simulink subsystem "Lateral_Position_Control"  (R2021b)
settings: Solver=VariableStepAuto  StartTime=0.0  StopTime=10.0  RelTol=1e-3
undefined symbols (not defined in the file or in its folder): IC0, md, md0, PredictionHorizon, Ts, XRef, YawRef, YRef
libraries: simulink_extras x5, mpcadaslib x1, cstblocks x1
settings Model: Creator=gabep  LastModifiedBy=gabep

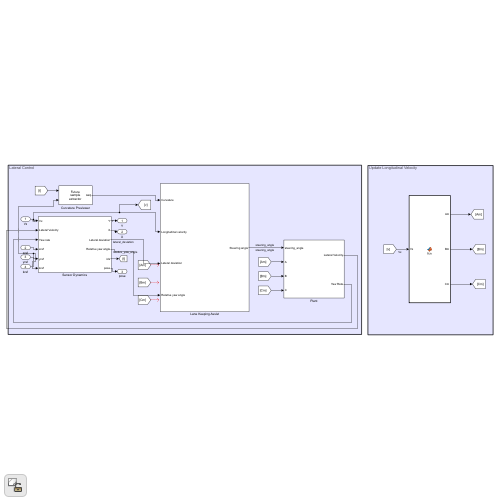
[thumbnail: Simulink's stored preview of the top-level diagram]
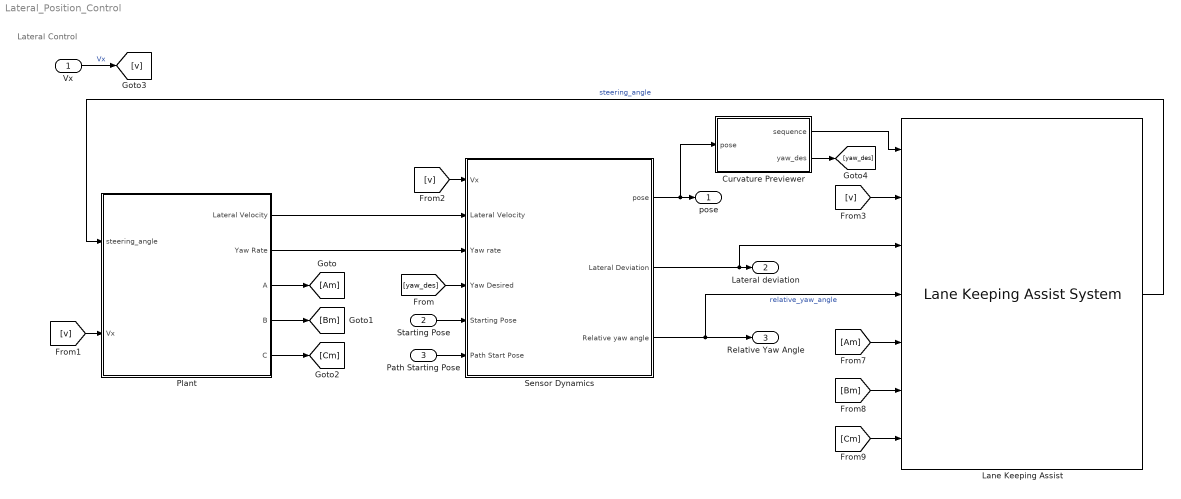
== system Lateral_Position_Control ==
  note: Lateral Control
  Vx : Inport
  Starting Pose : Inport  Port=2
  Path Starting Pose : Inport  Port=3
  Curvature Previewer : Subsystem  mask{signal=md, ts=Ts, steps=PredictionHorizon}
      mask prompts: signal "Signal name"; ts "Sampling time"; steps "Number of previewing steps"
      mask init:
      | ts = evalin('base',get_param(gcbh,'ts'));
      | signal = evalin('base',get_param(gcbh,'signal'));
      | steps = evalin('base',get_param(gcbh,'steps'));
      | data = mpc_previewer_maskinit(signal,ts);
      mask Display:
      | fprintf('Future\nsample\nextractor');
      | port_label('output', 1, 'seq')
      | %port_label('output', 2, '@t')
  Lane Keeping Assist : mpcadaslib/Lane Keeping Assist System  ModelType=Use vehicle model  VehicleMass=9053  VehicleYawInertia=52161  LengthToFront=2.7  LengthToRear=4.02  FrontTireStiffness=15000  RearTireStiffness=121000  EgoModelMatrixA=A  EgoModelMatrixB=B  EgoModelMatrixC=C  InitialLongVel=Vx0  TransportLag=0  MinSteering=u_min  umin_ext=off  MaxSteering=u_max  umax_ext=off  Ts=Ts  PredictionHorizon=PredictionHorizon  ControllerBehavior=0.500  suboptimal=off  maxiter=10  datatypeopt=double  optmode=off  trackmode=off
      settings: SourceProductBaseCode=MP
  Plant : Subsystem
  Sensor Dynamics : Subsystem
  pose : Outport
  Lateral deviation : Outport  Port=2
  Relative Yaw Angle : Outport  Port=3
  wires:
  Plant/2(Yaw Rate) -> Sensor Dynamics/3(Yaw rate)
  Plant/1(Lateral Velocity) -> Sensor Dynamics/2(Lateral Velocity)
  [Am] -> Lane Keeping Assist/5
  [Bm] -> Lane Keeping Assist/6
  [Cm] -> Lane Keeping Assist/7
  Sensor Dynamics/3(Relative yaw angle) -> Relative Yaw Angle/1, Lane Keeping Assist/4  "relative_yaw_angle"
  Lane Keeping Assist/1 -> Plant/1(steering_angle)  "steering_angle"
  Plant/3(A) -> [Am]
  Plant/5(C) -> [Cm]
  Plant/4(B) -> [Bm]
  Starting Pose/1 -> Sensor Dynamics/5(Starting Pose)
  Curvature Previewer/1(sequence) -> Lane Keeping Assist/1
  Path Starting Pose/1 -> Sensor Dynamics/6(Path Start Pose)
  Sensor Dynamics/1(pose) -> Curvature Previewer/1(pose), pose/1
  Vx/1 -> [v]  "Vx"
  [v] -> Sensor Dynamics/1(Vx)
  [v] -> Lane Keeping Assist/2
  [v] -> Plant/2(Vx)
  Curvature Previewer/2(yaw_des) -> [yaw_des]
  [yaw_des] -> Sensor Dynamics/4(Yaw Desired)
  Sensor Dynamics/2(Lateral Deviation) -> Lateral deviation/1, Lane Keeping Assist/3

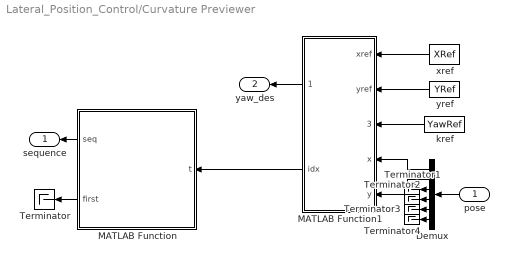
== system Lateral_Position_Control/Curvature Previewer ==
  pose : Inport
  Demux : Demux  Outputs=6
  MATLAB Function : MATLAB Function  TreatAsAtomicUnit=on
  MATLAB Function1 : MATLAB Function  TreatAsAtomicUnit=on
  Terminator{,1..4} (5 alike) : Terminator
  kref : Constant  Value=YawRef
  xref : Constant  Value=XRef
  yref : Constant  Value=YRef
  sequence : Outport  VectorParamsAs1DForOutWhenUnconnected=off
  yaw_des : Outport  Port=2
  wires:
  MATLAB Function1/1(yaw_des) -> yaw_des/1
  Demux/6 -> Terminator4/1
  Demux/5 -> Terminator3/1
  Demux/4 -> Terminator2/1
  Demux/3 -> Terminator1/1
  Demux/2 -> MATLAB Function1/5(y)
  Demux/1 -> MATLAB Function1/4(x)
  pose/1 -> Demux/1
  kref/1 -> MATLAB Function1/3(yawref)
  yref/1 -> MATLAB Function1/2(yref)
  xref/1 -> MATLAB Function1/1(xref)
  MATLAB Function1/2(idx) -> MATLAB Function/1(t)
  MATLAB Function/2(first) -> Terminator/1
  MATLAB Function/1(seq) -> sequence/1

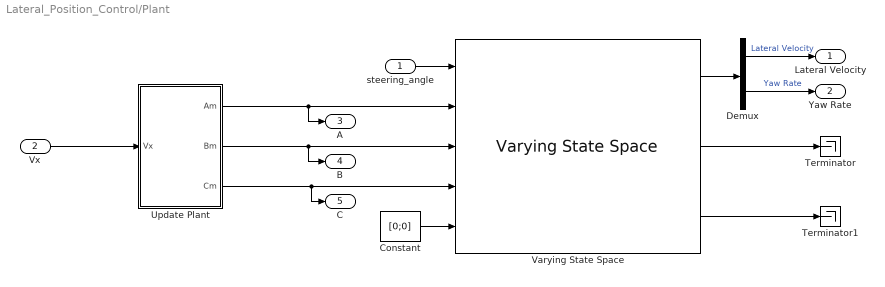
== system Lateral_Position_Control/Plant ==
  steering_angle : Inport
  Vx : Inport  Port=2
  Constant : Constant  Value=[0;0]
  Demux : Demux  Outputs=2
  Terminator : Terminator
  Terminator1 : Terminator
  Update Plant : MATLAB Function  TreatAsAtomicUnit=on
  Varying State Space : cstblocks/Linear Parameter Varying/Varying State Space  x0=0  xNames=''  OutputX=on  OutputDX=on
  Lateral Velocity : Outport
  Yaw Rate : Outport  Port=2
  A : Outport  Port=3
  B : Outport  Port=4
  C : Outport  Port=5
  wires:
  Vx/1 -> Update Plant/1(Vx)
  Update Plant/3(Cm) -> Varying State Space/4, C/1
  Update Plant/1(Am) -> Varying State Space/2, A/1
  Update Plant/2(Bm) -> Varying State Space/3, B/1
  Demux/2 -> Yaw Rate/1  "Yaw Rate"
  Varying State Space/1 -> Demux/1
  Varying State Space/2 -> Terminator/1
  Demux/1 -> Lateral Velocity/1  "Lateral Velocity"
  Varying State Space/3 -> Terminator1/1
  Constant/1 -> Varying State Space/5
  steering_angle/1 -> Varying State Space/1

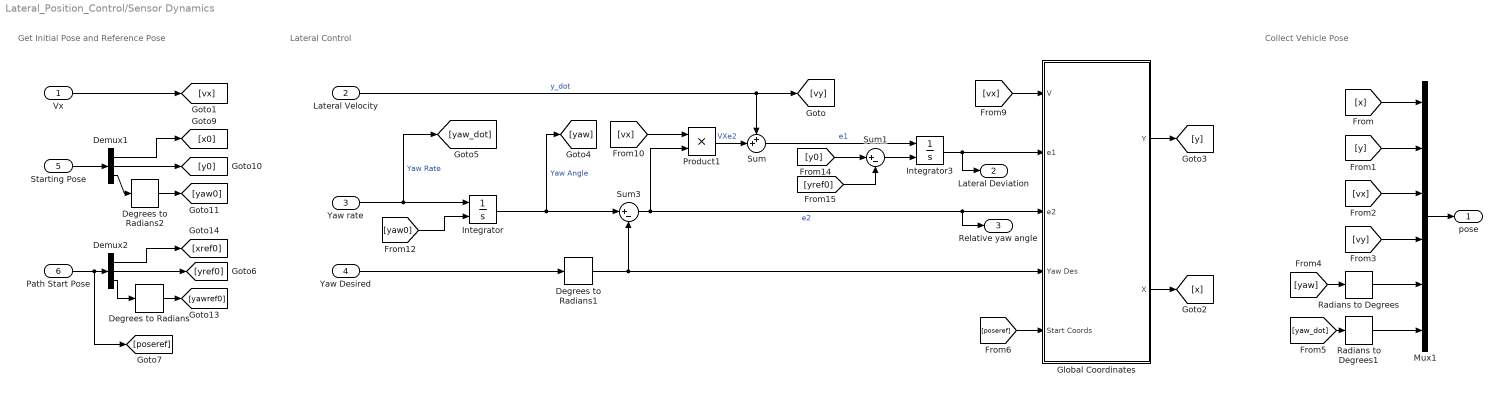
== system Lateral_Position_Control/Sensor Dynamics ==
  note: Get Initial Pose and Reference Pose
  note: Lateral Control
  note: Collect Vehicle Pose
  Vx : Inport
  Lateral Velocity : Inport  Port=2
  Yaw rate : Inport  Port=3
  Yaw Desired : Inport  Port=4
  Starting Pose : Inport  Port=5
  Path Start Pose : Inport  Port=6
  " Global Coordinates" : Subsystem
  Degrees to Radians : simulink_extras/Transformations/Degrees to Radians
  Degrees to Radians1 : simulink_extras/Transformations/Degrees to Radians
  Degrees to Radians2 : simulink_extras/Transformations/Degrees to Radians
  Demux1 : Demux  Outputs=3
  Demux2 : Demux  Outputs=3
  Integrator : Integrator  InitialConditionSource=external  InitialCondition=IC0.yaw_angle0
  Integrator3 : Integrator  InitialConditionSource=external  InitialCondition=IC0.y0 - md0.y(130)
  Mux1 : Mux  Inputs=6
  Product1 : Product
  Radians to Degrees : simulink_extras/Transformations/Radians to Degrees
  Radians to Degrees1 : simulink_extras/Transformations/Radians to Degrees
  Sum : Sum  Inputs=++|
  Sum1 : Sum  Inputs=|+-
  Sum3 : Sum  Inputs=|+-
  pose : Outport
  Lateral Deviation : Outport  Port=2
  Relative yaw angle : Outport  Port=3  VectorParamsAs1DForOutWhenUnconnected=off
  wires:
  Degrees to Radians1/1 -> " Global Coordinates"/4(Yaw Des), Sum3/2
  Yaw Desired/1 -> Degrees to Radians1/1
  Path Start Pose/1 -> Demux2/1, [poseref]
  Degrees to Radians2/1 -> [yaw0]
  Radians to Degrees/1 -> Mux1/5
  [vx] -> " Global Coordinates"/1(V)
  Degrees to Radians/1 -> [yawref0]
  [poseref] -> " Global Coordinates"/5(Start Coords)
  Demux2/2 -> [yref0]
  Demux2/1 -> [xref0]
  Sum1/1 -> Integrator3/2
  Sum/1 -> Integrator3/1  "e1"
  [yref0] -> Sum1/2
  [y0] -> Sum1/1
  [yaw0] -> Integrator/2
  [vx] -> Product1/1
  Vx/1 -> [vx]
  Demux2/3 -> Degrees to Radians/1
  Demux1/2 -> [y0]
  Demux1/3 -> Degrees to Radians2/1
  Demux1/1 -> [x0]
  Starting Pose/1 -> Demux1/1
  [yaw] -> Radians to Degrees/1
  [yaw_dot] -> Radians to Degrees1/1
  [vy] -> Mux1/4
  Mux1/1 -> pose/1
  [x] -> Mux1/1
  Radians to Degrees1/1 -> Mux1/6
  [vx] -> Mux1/3
  [y] -> Mux1/2
  Integrator3/1 -> " Global Coordinates"/2(e1), Lateral Deviation/1
  Sum3/1 -> " Global Coordinates"/3(e2), Relative yaw angle/1, Product1/2  "e2"
  " Global Coordinates"/2(X) -> [x]
  " Global Coordinates"/1(Y) -> [y]
  Product1/1 -> Sum/2  "VXe2"
  Lateral Velocity/1 -> [vy], Sum/1  "y_dot"
  Integrator/1 -> [yaw], Sum3/1  "Yaw Angle"
  Yaw rate/1 -> Integrator/1, [yaw_dot]  "Yaw Rate"

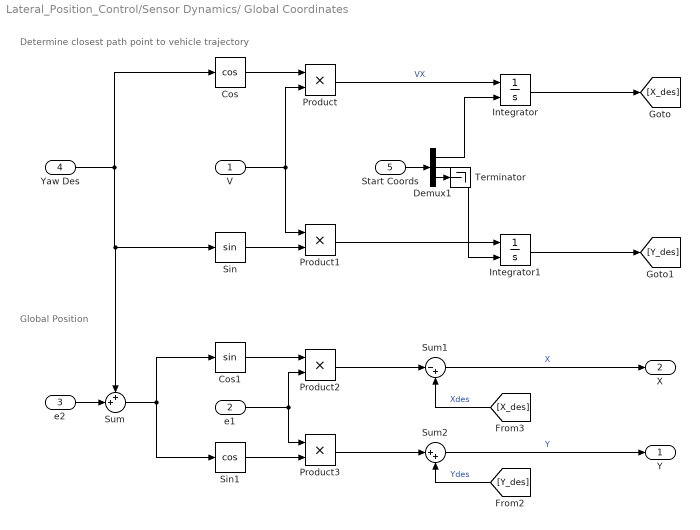
== system Lateral_Position_Control/Sensor Dynamics/ Global Coordinates ==
  note: Global Position
  note: Determine closest path point to vehicle trajectory
  V : Inport
  e1 : Inport  Port=2
  e2 : Inport  Port=3
  Yaw Des : Inport  Port=4
  Start Coords : Inport  Port=5
  Cos : Trigonometry  Operator=cos
  Cos1 : Trigonometry
  Demux1 : Demux  Outputs=3
  Integrator : Integrator  InitialConditionSource=external  InitialCondition=md0.x(130)
  Integrator1 : Integrator  InitialConditionSource=external  InitialCondition=md0.y(130)
  Product{,1..3} (4 alike) : Product
  Sin : Trigonometry
  Sin1 : Trigonometry  Operator=cos
  Sum : Sum  Inputs=++|
  Sum1 : Sum  Inputs=|-+
  Sum2 : Sum  Inputs=|++
  Terminator : Terminator
  Y : Outport
  X : Outport  Port=2
  wires:
  [X_des] -> Sum1/2  "Xdes"
  Sum1/1 -> X/1  "X"
  Sum2/1 -> Y/1  "Y"
  [Y_des] -> Sum2/2  "Ydes"
  Cos/1 -> Product/1
  Product1/1 -> Integrator1/1
  Yaw Des/1 -> Sin/1, Sum/1, Cos/1
  Product/1 -> Integrator/1  "VX"
  Demux1/3 -> Terminator/1
  Demux1/2 -> Integrator1/2
  Demux1/1 -> Integrator/2
  Start Coords/1 -> Demux1/1
  Integrator1/1 -> [Y_des]
  Integrator/1 -> [X_des]
  V/1 -> Product1/1, Product/2
  Sin/1 -> Product1/2
  Product3/1 -> Sum2/1
  Product2/1 -> Sum1/1
  e1/1 -> Product3/1, Product2/2
  Sum/1 -> Cos1/1, Sin1/1
  Sin1/1 -> Product3/2
  Cos1/1 -> Product2/1
  e2/1 -> Sum/2

== matlab function Lateral_Position_Control/Curvature Previewer/MATLAB Function ==
  settings: updateMethod=DISCRETE  sampleTime=ts
  data: data parameter; seq output; steps parameter; t input; first output
function [seq, first] = fcn(data, steps, t)
[seq,first,~] = mpcblock_preview('md',data,steps,t);

== matlab function Lateral_Position_Control/Curvature Previewer/MATLAB Function1 ==
  data: xref input; yref input; yawref input; x input; y input; yaw_des output; idx output
function [yaw_des, idx] = fcn(xref, yref, yawref, x, y)

d = pdist2([x,y],[xref yref]);
[~, i]= mink(d,1);
idx=i(1);

yaw_des = mean(yawref(i));

== matlab function Lateral_Position_Control/Plant/Update Plant ==
  data: Vx input; Am output; Bm output; Cm output
function [Am, Bm, Cm] = fcn(Vx)
    [Am,Bm,Cm] = truck_trailer_model(Vx);
end
